simulink model "Sub3_2023"  (R2023b)
settings: Solver=FixedStepDiscrete  StartTime=0.0  StopTime=4.5  FixedStep=75e-6  RelTol=1e-3  EnableMultiTasking=on
undefined symbols (not defined in the file or in its folder): D1, D11, Delta
libraries: spsSeriesRLCBranchLib x41, spsLoadFlowBusLib x29, spsDistributedParametersLineLib x19, spsThreePhaseSeriesRLCLoadLib x15, spsThreePhaseTransformerTwoWindingsLib x13, spsThreePhaseParallelRLCLoadLib x11, spsThreePhaseVIMeasurementLib x11, spsSynchronousMachinepuStandardLib x7, spsExcitationSystemLib x7, spsHydraulicTurbineandGovernorLib x7, spsGenericPowerSystemStabilizerLib x7, spsMultiBandPowerSystemStabilizerLib x7
(part 5 of 5)

== system Sub3_2023/Sub3/North-West Network2/Regulators2/Turbine  & Excitation Regulators/Stabilisateur ==
  Pm : Inport
  Pe : Inport  Port=2
  dw : Inport  Port=3
  Generic Power System Stabilizer : spsGenericPowerSystemStabilizerLib/Generic Power System Stabilizer  Tsensor=15e-3  K=2.5  Twashout=1  Tleadlag1="[0.06  1]"  Tleadlag2="[0  0]"  VSlimits=[-0.15 0.15]  Vinit=0  Plot_On=off  MagdB_On=on  FreqRange=logspace(-2,2,500)
      settings: LibrarySourceBlock=|
      | sps_lib/Electrical Machines/Synchronous Machine Control/Generic
      | Power System Stabilizer
  Ground1 : Ground
  Multi-Band Power System Stabilizer : spsMultiBandPowerSystemStabilizerLib/Multi-Band Power System Stabilizer  OperationMode=Simplified settings  Kg=0.7  GL=[0.2 10]  GI=[0.9 30]  GH=[12.0 115]  GLd=[66 66 9.4]  TcLF=[1.667 2 0 0 0 0 2 2.4 0 0 0 0 1 1]  GId=[66 66 47.6]  TcIF=[1 1 0.25 0.3 0 0 1 1 0.3 0.36 0 0 0 0]  GHd=[66 66 233]  TcHF="[0.01 0.012 0 0 0 0  0.012 0.0144 0 0 0 0 1 1]"  LIM=[.075 .15 .15 .15]  Plot_On=off  MagdB_On=on  FreqRange=logspace(-2,2,500)
      settings: LibrarySourceBlock=|
      | sps_lib/Electrical Machines/Synchronous Machine Control/Multi-Band
      | Power System Stabilizer
  Multiport Switch : MultiPortSwitch
  Sum2 : Sum  Inputs=+-  InputSameDT=on  SaturateOnIntegerOverflow=on  OutDataTypeStr=Inherit: Same as first input
  Stab : Outport  InitialOutput=0  VectorParamsAs1DForOutWhenUnconnected=off
  wires:
  dw/1 -> Multi-Band Power System Stabilizer/1
  [PSS_select_3] -> Multiport Switch/1
  Ground1/1 -> Multiport Switch/2
  Pe/1 -> Sum2/2
  Pm/1 -> Sum2/1
  Sum2/1 -> Generic Power System Stabilizer/1
  Generic Power System Stabilizer/1 -> Multiport Switch/3
  Multiport Switch/1 -> Stab/1
  Multi-Band Power System Stabilizer/1 -> Multiport Switch/4

== system Sub3_2023/Sub3/North-West Network2/Regulators3/Turbine  & Excitation Regulators/Stabilisateur ==
  Pm : Inport
  Pe : Inport  Port=2
  dw : Inport  Port=3
  Generic Power System Stabilizer : spsGenericPowerSystemStabilizerLib/Generic Power System Stabilizer  Tsensor=15e-3  K=2.5  Twashout=1  Tleadlag1="[0.06  1]"  Tleadlag2="[0  0]"  VSlimits=[-0.15 0.15]  Vinit=0  Plot_On=off  MagdB_On=on  FreqRange=logspace(-2,2,500)
      settings: LibrarySourceBlock=|
      | sps_lib/Electrical Machines/Synchronous Machine Control/Generic
      | Power System Stabilizer
  Ground1 : Ground
  Multi-Band Power System Stabilizer : spsMultiBandPowerSystemStabilizerLib/Multi-Band Power System Stabilizer  OperationMode=Simplified settings  Kg=0.7  GL=[0.2 10]  GI=[0.9 30]  GH=[12.0 115]  GLd=[66 66 9.4]  TcLF=[1.667 2 0 0 0 0 2 2.4 0 0 0 0 1 1]  GId=[66 66 47.6]  TcIF=[1 1 0.25 0.3 0 0 1 1 0.3 0.36 0 0 0 0]  GHd=[66 66 233]  TcHF="[0.01 0.012 0 0 0 0  0.012 0.0144 0 0 0 0 1 1]"  LIM=[.075 .15 .15 .15]  Plot_On=off  MagdB_On=on  FreqRange=logspace(-2,2,500)
      settings: LibrarySourceBlock=|
      | sps_lib/Electrical Machines/Synchronous Machine Control/Multi-Band
      | Power System Stabilizer
  Multiport Switch : MultiPortSwitch
  Sum2 : Sum  Inputs=+-  InputSameDT=on  SaturateOnIntegerOverflow=on  OutDataTypeStr=Inherit: Same as first input
  Stab : Outport  InitialOutput=0  VectorParamsAs1DForOutWhenUnconnected=off
  wires:
  Multiport Switch/1 -> Stab/1
  Generic Power System Stabilizer/1 -> Multiport Switch/3
  Sum2/1 -> Generic Power System Stabilizer/1
  Pm/1 -> Sum2/1
  Pe/1 -> Sum2/2
  Ground1/1 -> Multiport Switch/2
  [PSS_select_3] -> Multiport Switch/1
  dw/1 -> Multi-Band Power System Stabilizer/1
  Multi-Band Power System Stabilizer/1 -> Multiport Switch/4

== system Sub3_2023/Sub3/North-West Network2/Regulators4/Turbine  & Excitation Regulators/Stabilisateur ==
  Pm : Inport
  Pe : Inport  Port=2
  dw : Inport  Port=3
  Generic Power System Stabilizer : spsGenericPowerSystemStabilizerLib/Generic Power System Stabilizer  Tsensor=15e-3  K=2.5  Twashout=1  Tleadlag1="[0.06  1]"  Tleadlag2="[0  0]"  VSlimits=[-0.15 0.15]  Vinit=0  Plot_On=off  MagdB_On=on  FreqRange=logspace(-2,2,500)
      settings: LibrarySourceBlock=|
      | sps_lib/Electrical Machines/Synchronous Machine Control/Generic
      | Power System Stabilizer
  Ground1 : Ground
  Multi-Band Power System Stabilizer : spsMultiBandPowerSystemStabilizerLib/Multi-Band Power System Stabilizer  OperationMode=Simplified settings  Kg=0.7  GL=[0.2 10]  GI=[0.9 30]  GH=[12.0 115]  GLd=[66 66 9.4]  TcLF=[1.667 2 0 0 0 0 2 2.4 0 0 0 0 1 1]  GId=[66 66 47.6]  TcIF=[1 1 0.25 0.3 0 0 1 1 0.3 0.36 0 0 0 0]  GHd=[66 66 233]  TcHF="[0.01 0.012 0 0 0 0  0.012 0.0144 0 0 0 0 1 1]"  LIM=[.075 .15 .15 .15]  Plot_On=off  MagdB_On=on  FreqRange=logspace(-2,2,500)
      settings: LibrarySourceBlock=|
      | sps_lib/Electrical Machines/Synchronous Machine Control/Multi-Band
      | Power System Stabilizer
  Multiport Switch : MultiPortSwitch
  Sum2 : Sum  Inputs=+-  InputSameDT=on  SaturateOnIntegerOverflow=on  OutDataTypeStr=Inherit: Same as first input
  Stab : Outport  InitialOutput=0  VectorParamsAs1DForOutWhenUnconnected=off
  wires:
  dw/1 -> Multi-Band Power System Stabilizer/1
  [PSS_select_3] -> Multiport Switch/1
  Ground1/1 -> Multiport Switch/2
  Pe/1 -> Sum2/2
  Pm/1 -> Sum2/1
  Sum2/1 -> Generic Power System Stabilizer/1
  Generic Power System Stabilizer/1 -> Multiport Switch/3
  Multiport Switch/1 -> Stab/1
  Multi-Band Power System Stabilizer/1 -> Multiport Switch/4

== system Sub3_2023/Sub3/North_East Network2/Regulateurs6/Turbine  & Excitation Regulators/Stabilisateur ==
  Pm : Inport
  Pe : Inport  Port=2
  dw : Inport  Port=3
  Generic Power System Stabilizer : spsGenericPowerSystemStabilizerLib/Generic Power System Stabilizer  Tsensor=15e-3  K=2.5  Twashout=1  Tleadlag1="[0.06  1]"  Tleadlag2="[0  0]"  VSlimits=[-0.15 0.15]  Vinit=0  Plot_On=off  MagdB_On=on  FreqRange=logspace(-2,2,500)
      settings: LibrarySourceBlock=|
      | sps_lib/Electrical Machines/Synchronous Machine Control/Generic
      | Power System Stabilizer
  Ground1 : Ground
  Multi-Band Power System Stabilizer : spsMultiBandPowerSystemStabilizerLib/Multi-Band Power System Stabilizer  OperationMode=Simplified settings  Kg=0.7  GL=[0.2 10]  GI=[0.9 30]  GH=[12.0 115]  GLd=[66 66 9.4]  TcLF=[1.667 2 0 0 0 0 2 2.4 0 0 0 0 1 1]  GId=[66 66 47.6]  TcIF=[1 1 0.25 0.3 0 0 1 1 0.3 0.36 0 0 0 0]  GHd=[66 66 233]  TcHF="[0.01 0.012 0 0 0 0  0.012 0.0144 0 0 0 0 1 1]"  LIM=[.075 .15 .15 .15]  Plot_On=off  MagdB_On=on  FreqRange=logspace(-2,2,500)
      settings: LibrarySourceBlock=|
      | sps_lib/Electrical Machines/Synchronous Machine Control/Multi-Band
      | Power System Stabilizer
  Multiport Switch : MultiPortSwitch
  Sum2 : Sum  Inputs=+-  InputSameDT=on  SaturateOnIntegerOverflow=on  OutDataTypeStr=Inherit: Same as first input
  Stab : Outport  InitialOutput=0  VectorParamsAs1DForOutWhenUnconnected=off
  wires:
  Multiport Switch/1 -> Stab/1
  Generic Power System Stabilizer/1 -> Multiport Switch/3
  Sum2/1 -> Generic Power System Stabilizer/1
  Pm/1 -> Sum2/1
  Pe/1 -> Sum2/2
  Ground1/1 -> Multiport Switch/2
  [PSS_select_3] -> Multiport Switch/1
  dw/1 -> Multi-Band Power System Stabilizer/1
  Multi-Band Power System Stabilizer/1 -> Multiport Switch/4

== system Sub3_2023/Sub3/North_East Network2/Regulateurs7/Turbine  & Excitation Regulators/Stabilisateur ==
  Pm : Inport
  Pe : Inport  Port=2
  dw : Inport  Port=3
  Generic Power System Stabilizer : spsGenericPowerSystemStabilizerLib/Generic Power System Stabilizer  Tsensor=15e-3  K=2.5  Twashout=1  Tleadlag1="[0.06  1]"  Tleadlag2="[0  0]"  VSlimits=[-0.15 0.15]  Vinit=0  Plot_On=off  MagdB_On=on  FreqRange=logspace(-2,2,500)
      settings: LibrarySourceBlock=|
      | sps_lib/Electrical Machines/Synchronous Machine Control/Generic
      | Power System Stabilizer
  Ground1 : Ground
  Multi-Band Power System Stabilizer : spsMultiBandPowerSystemStabilizerLib/Multi-Band Power System Stabilizer  OperationMode=Simplified settings  Kg=0.7  GL=[0.2 10]  GI=[0.9 30]  GH=[12.0 115]  GLd=[66 66 9.4]  TcLF=[1.667 2 0 0 0 0 2 2.4 0 0 0 0 1 1]  GId=[66 66 47.6]  TcIF=[1 1 0.25 0.3 0 0 1 1 0.3 0.36 0 0 0 0]  GHd=[66 66 233]  TcHF="[0.01 0.012 0 0 0 0  0.012 0.0144 0 0 0 0 1 1]"  LIM=[.075 .15 .15 .15]  Plot_On=off  MagdB_On=on  FreqRange=logspace(-2,2,500)
      settings: LibrarySourceBlock=|
      | sps_lib/Electrical Machines/Synchronous Machine Control/Multi-Band
      | Power System Stabilizer
  Multiport Switch : MultiPortSwitch
  Sum2 : Sum  Inputs=+-  InputSameDT=on  SaturateOnIntegerOverflow=on  OutDataTypeStr=Inherit: Same as first input
  Stab : Outport  InitialOutput=0  VectorParamsAs1DForOutWhenUnconnected=off
  wires:
  dw/1 -> Multi-Band Power System Stabilizer/1
  [PSS_select_3] -> Multiport Switch/1
  Ground1/1 -> Multiport Switch/2
  Pe/1 -> Sum2/2
  Pm/1 -> Sum2/1
  Sum2/1 -> Generic Power System Stabilizer/1
  Generic Power System Stabilizer/1 -> Multiport Switch/3
  Multiport Switch/1 -> Stab/1
  Multi-Band Power System Stabilizer/1 -> Multiport Switch/4
